simulink library "cm_custom"  (R2018b)
settings: Solver=VariableStepAuto  StartTime=0.0  StopTime=10.0  RelTol=1e-3
undefined symbols (not defined in the file or in its folder): DiscIntNeverNeededParam
libraries: simulink x19, raspberrypilib x4, $bdroot x2, speedgoatlib_fpga x2, androidcommunicationlib x1, embdlinuxlib x1, commutil2 x1
(part 1 of 2)
settings Model: Creator=carlosma  LastModifiedBy=Raymond
settings DebuggingCC: LibraryContextMissingDiagnostic=none
settings SFSimCC: SimUserLibraries=datatypes.h  SimUseLocalCustomCode=off
settings RTWCC: RTWUseLocalCustomCode=off  RTWUseSimCustomCode=on  CustomLibrary=datatypes.h  TargetLang=C++
settings GRTTargetCC: TargetLangStandard=C++03 (ISO)  MultiInstanceERTCode=on  CodeInterfacePackaging=C++ class

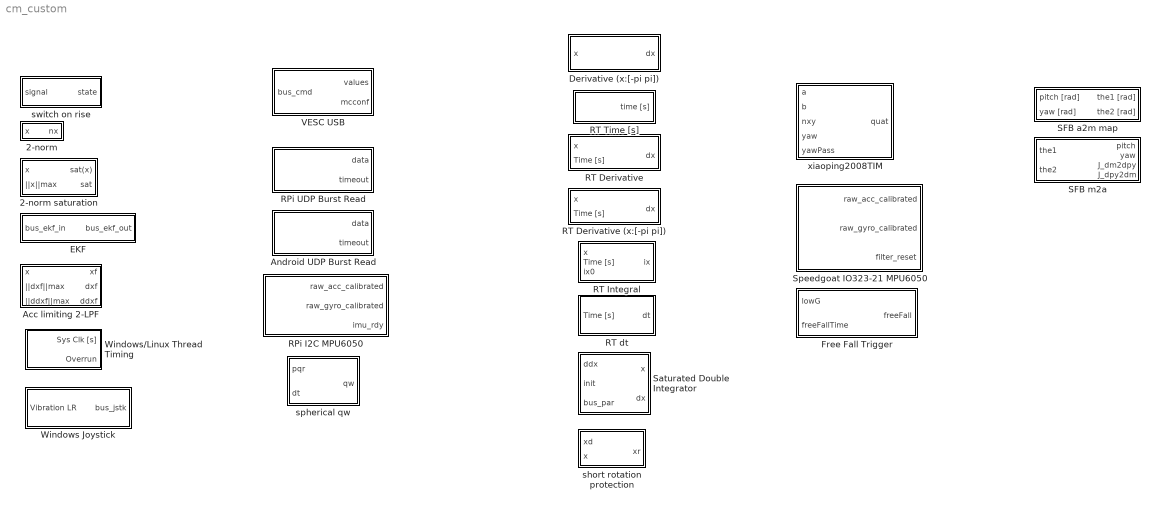
== system cm_custom ==
  2-norm : Subsystem  mask(Vector 2-norm){}
      mask help:
      | Computes vector 2-norm.
      |
      | ---
      | CMA 18DEC18
  2-norm saturation : Subsystem  mask(2-norm saturation){}
      mask help:
      | Saturates the input when its vector 2-norm reaches the defined limit.
      |
      | Maintains vector direction.
      |
      | ---
      | CMA 18DEC18
  Acc limiting 2-LPF : Subsystem  TreatAsAtomicUnit=on  SystemSampleTime=PAR_SMPLT  mask(Critically damped 2nd order LPF with acceleration and velocity limit){PAR_SMPLT=-1}
      mask prompts: PAR_SMPLT "Sampling Time [s]"
      mask help:
      | Limits are applied on the norms of the respective signals to retain signal directions.
      |
      | ddxf = -2*k*(xf - x) - k^2 * dxf;
      |
      | ||ddxf|| <= k^2 * ||xf - x|| + 2*k * ||dxf|| := ||ddxf||max
      | => k^2 * ||xf - x|| + k * 2 * ||dxf|| - ||ddxf||max = 0
      | => k = (-2*||dxf|| + sqrt(4*||dxf||^2 + 4 * ||xf - x|| * ||ddxf||max)) / (2 * ||xf - x|| + 1e-3); // norm division safe
      |
      | // satdxf not proven
  Android UDP Burst Read : Subsystem  TreatAsAtomicUnit=on  SystemSampleTime=PAR_SMPLT  mask(Android UDP Burst Read){PAR_LOCAL_IP_PORT=24001, PAR_BYTES_PER_PACKET=9, PAR_NBURST=100, PAR_TIMEOUT_TIME=1, PAR_SMPLT=0.1}
      mask prompts: PAR_LOCAL_IP_PORT "Local IP port"; PAR_BYTES_PER_PACKET "Expected nbytes per packet"; PAR_NBURST "Maximum burst read number"; PAR_TIMEOUT_TIME "Timeout after [s]"; PAR_SMPLT "Sampling Time [s]"
      mask help:
      | An extension to the official UDP read block.
      |
      | Supports burst reads and timeout detection.
      |
      | REQUIRES the official Simulink Android support package (2018b+).
      |
      | ---
      | Tested on a Samsung A9, Anrdroid 8.0.
      | Usable in External mode.
      | Embedded Coder safe.
      |
      | ---
      | CMA 8MAR2019
  Derivative (x:[-pi pi]) : Subsystem  TreatAsAtomicUnit=on  mask(RT Derivative (x:[-pi pi])){}
      mask help:
      | Computes the time derivative of the input using RT Time with x being an angular state between -pi and pi (matrix inputs are accepted).
      |
      | Requires one instance of the RT Time block.
      |
      | ---
      | Tested on Windows 10, Raspbian.
      | Usable in Simulation and External mode.
      | Embedded Coder safe.
      |
      | ---
      | CMA 14FEB19
  EKF : Subsystem  mask(EKF/LKF block){}
      mask help:
      | One step EKF computation for smooth nonlinear plants with continuous states.
      |
      | // Subscript 'o' means OLD
      | Smooth nonlinear plant with white process and measurement noises (wo, v)
      | x = f(xo, uo) + wo
      | y = g(x) + v
      |
      | bus_ekf_in signals
      | fuse // flag to activate or omit fusion
      | xh = f(xho, uo) // estimated mean
      | yh = g(xh) // estimated measurement
      | y // current measurement
      | A = df/dx | xo,uo // Jacobian A
      | B = df/du | xo,uo // Jacobian B
      | C = dg/dx | xh // Jacobian C
      | Qo = cov(wo) // process noise covariance
      | R = cov(v) // measurement noise covariance
      | Po = cov(xo-xho) // old mean covariance
      |
      | bus_ekf_out signals
      | x // filtered state mean
      | P // filtered state covariance
  Free Fall Trigger : Stateflow chart  TreatAsAtomicUnit=on
  RPi I2C MPU6050 : Stateflow chart  TreatAsAtomicUnit=on  SystemSampleTime=PAR_SMPLT  mask{PAR_SENS_ACC=([10.47 9.783 10.1] - [-9.234 -9.837 -9.396]) / 2 / 8192, PAR_SENS_GYRO=[1 1 1] * pi / 180 / 16.4, PAR_OFFSET_ACC=-[0.5758 -0.02694 0.673], PAR_OFFSET_GYRO=-[-0.133 -0.043 -0.023], PAR_SMPLT=0.001}
      mask prompts: PAR_SENS_ACC "Accelerometer sensitivities xyz [ms^-2/LSB]"; PAR_SENS_GYRO "Gyroscope sensitivities xyz [rad/LSB]"; PAR_OFFSET_ACC "Accelerometer offset xyz [ms^-2]"; PAR_OFFSET_GYRO "Gyroscope offset xyz [rad]"; PAR_SMPLT "Sampling Time [s]"
  RPi UDP Burst Read : Subsystem  TreatAsAtomicUnit=on  SystemSampleTime=PAR_SMPLT  mask(RPi UDP Burst Read){PAR_LOCAL_IP_PORT=24000, PAR_BYTES_PER_PACKET=13, PAR_NBURST=100, PAR_TIMEOUT_TIME=1, PAR_SMPLT=0.1}
      mask prompts: PAR_LOCAL_IP_PORT "Local IP port"; PAR_BYTES_PER_PACKET "Expected nbytes per packet"; PAR_NBURST "Maximum burst read number"; PAR_TIMEOUT_TIME "Timeout after [s]"; PAR_SMPLT "Sampling Time [s]"
      mask help:
      | An extension to the official UDP read block.
      |
      | Supports burst reads and timeout detection.
      |
      | REQUIRES the official Simulink Raspberry Pi support package (2018b+).
      |
      | ---
      | Tested on Raspbian.
      | Usable in External mode.
      | Embedded Coder safe.
      |
      | ---
      | CMA 8MAR2019
  RT Derivative : Subsystem  TreatAsAtomicUnit=on  mask(RT Derivative){}
      mask help:
      | Computes the time derivative of the input using RT Time.
      |
      | Requires one instance of the RT Time block.
      |
      | ---
      | Tested on Windows 10, Raspbian.
      | Usable in Simulation and External mode.
      | Embedded Coder safe.
      |
      | ---
      | CMA 14FEB19
  RT Derivative (x:[-pi pi]) : Subsystem  TreatAsAtomicUnit=on  mask(RT Derivative (x:[-pi pi])){}
      mask help:
      | Computes the time derivative of the input using RT Time with x being an angular state between -pi and pi (matrix inputs are accepted).
      |
      | Requires one instance of the RT Time block.
      |
      | ---
      | Tested on Windows 10, Raspbian.
      | Usable in Simulation and External mode.
      | Embedded Coder safe.
      |
      | ---
      | CMA 14FEB19
  RT Integral : Subsystem  TreatAsAtomicUnit=on  mask(RT Integral){PAR_SAT_UP=[inf], PAR_SAT_DOWN=[-inf]}
      mask prompts: PAR_SAT_UP "Upper integral saturation"; PAR_SAT_DOWN "Lower integral saturation"
      mask help:
      | Computes the time integral of the input using RT Time.
      |
      | Requires one instance of the RT Time block.
      |
      | ---
      | Tested on Windows 10, Raspbian.
      | Usable in Simulation and External mode.
      | Embedded Coder safe.
      |
      | ---
      | CMA 14FEB19
  RT Time [s] : Subsystem  mask(RT Time){}
      mask help:
      | Get RT time in seconds from <chrono>.
      |
      | ---
      | Tested on Windows 10, Raspbian.
      | Usable in Simulation.
      |
      | Link error on Windows external mode. - CMA 3APR19
      |
      | ---
      | CMA 3APR19
  RT dt : Subsystem  TreatAsAtomicUnit=on  mask(RT dt){}
      mask help:
      | Get last loop period using RT Time.
      |
      | Requires one instance of the RT Time block.
      |
      | ---
      | Tested on Windows 10, Raspbian.
      | Usable in Simulation and External mode.
      | Embedded Coder safe.
      |
      | ---
      | CMA 7MAR19
  SFB a2m map : Subsystem  mask(SFB M_a2m (YZX rotation)){par_r=0.05, par_w=0.05, par_yawMax=40*pi/180, par_pitchMax=90*pi/180}
      mask prompts: par_r "SFB bearing radius [m]"; par_w "SFB bearing width [m]"; par_yawMax "Maximum |yaw| [rad]"; par_pitchMax "Maximum |pitch| [rad]"
      mask help:
      | Maps yaw (psi) and pitch (the) angles of an SFB tail to the corresponding motor 1 and motor 2 angles.
      |
      | (Top view)
      |          T
      |          |
      |  M1   |    M2
      | (pitch up positive for both motors)
      |
      | thep = (the1 + the2) / 2;
      | thef = (the1 - the2) / 2;
      | the = thep;
      | tan(psi) = -2*r/w *sin(the_f);
      | |psi|_max = atan(2*r/w); // mechanical limit; will be used if superceded by the user limit
      |
      | ---
      | CMA 18DEC18
      mask init:
      | par_yawMax = min(par_yawMax, atan(2 * par_r / par_w));
  SFB m2a : MATLAB Function  TreatAsAtomicUnit=on
  Saturated Double Integrator : Subsystem  mask(Saturated Double Integrator){}
      mask help:
      | Second order integrator block with output and velocity saturations.
      |
      | ---
      | CMA 26MAR19
  Speedgoat IO323-21 MPU6050 : Stateflow chart  TreatAsAtomicUnit=on  SystemSampleTime=0.001  mask{PAR_SENS_ACC=[1 1 1] .* 9.80665 / 8192, PAR_SENS_GYRO=[1 1 1] * pi / 180 / 16.4, PAR_OFFSET_ACC=[-0.635 0.09 0.21], PAR_OFFSET_GYRO=[0.0462 0.0342 0.0261]}
      mask prompts: PAR_SENS_ACC "Accelerometer sensitivities xyz [ms^-2/LSB]"; PAR_SENS_GYRO "Gyroscope sensitivities xyz [rad/LSB]"; PAR_OFFSET_ACC "Accelerometer offset xyz [ms^-2]"; PAR_OFFSET_GYRO "Gyroscope offset xyz [rad]"
  VESC USB : Subsystem  InitFcn=load('vesc_usb_slx_buses.mat');  TreatAsAtomicUnit=on  SystemSampleTime=PAR_SMPLT  mask(VESC USB (Linux)){PAR_VESC_DEV='/dev/VESC_SFB_1', POS_KP=0.001, POS_KI=0, POS_KD=0.001, POS_KD_FIL=0.2, POS_DIV=1, CURR_MAX=20, CURR_MIN=-20, CURR_IN_MAX=20, CURR_IN_MIN=-20, CURR_ABS_MAX=20, PAR_SMPLT=0.05}
      mask prompts: PAR_VESC_DEV "VESC ID"; POS_KP "p_pid_kp"; POS_KI "p_pid_ki"; POS_KD "p_pid_kd"; POS_KD_FIL "p_pid_kd_filter"; POS_DIV "p_pid_ang_div"; CURR_MAX "l_current_max"; CURR_MIN "l_current_min"; CURR_IN_MAX "l_in_current_max"; CURR_IN_MIN "l_in_current_min"; CURR_ABS_MAX "l_abs_current_max"; PAR_SMPLT "Sampling Time [s]"
      mask help:
      | IO functions to and from a VESC via USB.
      | Drag and drop the same block for connecting to multiple VESC devices.
      |
      | --- SLX MASK
      | Allows the declaration of device name and R/W of some of the parameters of mcconfig.
      | ALWAYS READ mcconfig before WRITING.
      | Wrong mcconfig settings MAY DAMAGE your HW and brick your VESC.
      |
      | --- Compatible Firmware
      | 3.52, 3.53
      |
      | --- Compatible Hosts
      | Raspbian, Ubuntu 18.04.2 LTS.
      |
      | --- IO
      | bus_cmd: mode, pos_cmd, current_cmd
      | mode: [0 1 2 3 4] = [idle pos_PID read_mcconfig write_mcconfig current_ctrl]
      |
      | mc_values bus
      | mcconfig bus
      |
      | --- Fixing /DEV/ on Linux (assuming the device of interest is /dev/ttyUSB0)
      | CLI: udevadm info --name=/dev/ttyUSB0 --attribute-walk
      | mark down KERNEL and SUBSYSTEMS properties
      | e.g. KERNELS=="1-1.1.2", SUBSYSTEMS=="usb"
      | note that 1.1.2 in KERNELS means the second USB port
      | CLI: sudo nano /etc/udev/rules.d/99-USB_VESC.rules
      | add
      | KERNELS=="1-1.1.2", SUBSYSTEMS=="usb", SYMLINK+="VESC_SFB_1"
      | where "VESC_SFB_1" is the fixed desired USB device name.
      | Save, exit, reboot.
      | "VESC_SFB_1" is now fixed to USB port 2.
      |
      | ---
      | Usable in External mode.
      | Embedded Coder safe.
      |
      | ---
      | CMA 16MAY19
      mask init:
      | PAR_VESC_DEV = [PAR_VESC_DEV 0];
      mask DialogControl Control4 Prompt: mcconfig
      mask DialogControl Control2 Prompt: Fetch
      mask DialogControl Control2 Callback:
      | set_param(gcb+"/PAR_MASK_MODE", 'value', num2str(2));
      | 
      | rto = get_param(gcb+"/mcconfig_read_disp",'RuntimeObject');
      | while ~(rto.InputPort(1).Data(1))
      |     rto = get_param(gcb+"/mcconfig_read_disp",'RuntimeObject');
      |     pause(0.5);
      | end
      | 
      | rto = get_param(gcb+"/mcconfig_p_pid_disp",'RuntimeObject');
      | set_param(gcb, 'POS_KP', num2str(rto.InputPort(1).Data(1), 5));
      | set_param(gcb, 'POS_KI', num2str(rto.InputPort(1).Data(2), 5));
      | set_param(gcb, 'POS_KD', num2str(rto.InputPort(1).Data(3), 5));
      | set_param(gcb, 'POS_KD_FIL', num2str(rto.InputPort(1).Data(4), 5));
      | set_param(gcb, 'POS_DIV', num2str(rto.InputPort(1).Data(5), 5));
      | 
      | rto = get_param(gcb+"/mcconfig_current_lims_disp",'RuntimeObject');
      | set_param(gcb, 'CURR_MAX', num2str(rto.InputPort(1).Data(1), 5));
      | set_param(gcb, 'CURR_MIN', num2str(rto.InputPort(1).Data(2), 5));
      | set_param(gcb, 'CURR_IN_MAX', num2str(rto.InputPort(1).Data(3), 5));
      | set_param(gcb, 'CURR_IN_MIN', num2str(rto.InputPort(1).Data(4), 5));
      | set_param(gcb, 'CURR_ABS_MAX', num2str(rto.InputPort(1).Data(5), 5));
      | 
      | set_param(gcb+"/PAR_MASK_MODE", 'value', num2str(0));
      mask DialogControl Control3 Prompt: Write
      mask DialogControl Control3 Callback:
      | PID_PARAMS = [str2num(get_param(gcb, 'POS_KP')),...
      |               str2num(get_param(gcb, 'POS_KI')),...
      |               str2num(get_param(gcb, 'POS_KD')),...
      |               str2num(get_param(gcb, 'POS_KD_FIL')),...
      |               str2num(get_param(gcb, 'POS_DIV'))];
      | CURR_PARAMS = [str2num(get_param(gcb, 'CURR_MAX')),...
      |               str2num(get_param(gcb, 'CURR_MIN')),...
      |               str2num(get_param(gcb, 'CURR_IN_MAX')),...
      |               str2num(get_param(gcb, 'CURR_IN_MIN')),...
      |               str2num(get_param(gcb, 'CURR_ABS_MAX'))];
      | 
      | set_param(gcb+"/PAR_PID_GAINS", 'value', mat2str(PID_PARAMS));
      | set_param(gcb+"/PAR_CURR_LIMS", 'value', mat2str(CURR_PARAMS));
      | 
      | set_param(gcb+"/PAR_MASK_MODE", 'value', num2str(3)); % write mode
      | pause(0.5);
      | set_param(gcb+"/PAR_MASK_MODE", 'value', num2str(2)); % read mode
      | 
      | rto = get_param(gcb+"/mcconfig_read_disp",'RuntimeObject');
      | while ~(rto.InputPort(1).Data(1))
      |     rto = get_param(gcb+"/mcconfig_read_disp",'RuntimeObject');
      |     pause(0.5);
      | end
      | 
      | set_param(gcb+"/PAR_MASK_MODE", 'value', num2str(0));
  Windows Joystick : Subsystem  TreatAsAtomicUnit=on  SystemSampleTime=PAR_SMPLT  mask(Windows xinput joystick read){PAR_JSTKID=Joystick 1, PAR_SMPLT=0.05}
      mask prompts: PAR_JSTKID "Joystick ID"; PAR_SMPLT "Sampling Time [s]"
      mask help:
      | Tested on Windows 10 Enterprise Edition, x64, XBOX360 controller.
      | User can connect up to 4 controllers at the same time.
      |
      | This block can be used in both Normal and External modes.
      | Embedded Coder tolerant.
      |
      | Buttons [16]	[boolean]	[0 1]
      | LT RT 		[float] 		[-1 1]
      | LX LY RX RY	[float] 		[-1 1]
      | Connection 	[boolean]	[0 1]
      |
      | Vibration LR 	[float]		[0 1]
      |
      | ---
      | <windows.h>
      | <xinput.h>
      | #pragma comment(lib, "XInput.lib")
      |
      | ---
      | CMA 11DEC18
      mask init:
      | PAR_JSTKID = PAR_JSTKID - 1; % base zero
      mask TypeOptions PAR_JSTKID: Joystick 1 | Joystick 2 | Joystick 3 | Joystick 4
  Windows/Linux Thread Timing : Subsystem  TreatAsAtomicUnit=on  SystemSampleTime=PAR_SMPLT  mask(Thread Timing){PAR_SMPLT=1e-3}
      mask prompts: PAR_SMPLT "Thread base sampling time [s] (DO NOT USE -1)"
      mask help:
      | This block slows down the thread to close to real time.
      |
      | Tested on
      | - Windows 10 Enterprise Edition, x64,
      | - Ubuntu 18.04.2 LTS.
      |
      | This block can be used in both Normal and External Modes.
      |
      | Embedded Coder compatible.
      |
      | ---
      | #include<chrono>
      | #include<thread>
      |
      | ---
      | CMA 16MAY19
  short rotation protection : Subsystem  mask(Short Rotation Protection){PAR_MAX_XT=0.95*pi}
      mask prompts: PAR_MAX_XT "Maximum angular error (0,pi)"
      mask help:
      | This block ensures that the new commanded position will not cause an unwanted motor short rotation.
      |
      | The maximum angular error parameter X (<pi) ensures that the new reference angle would be at most X rad away from the current motor angle.
      |
      | e.g.
      | Without protection: if x = -150deg and xd = 150deg, a short short rotation of -60deg will occur downstream.
      | With protection: if x = -150deg and xd = 150deg, a proper rotation of +300deg will occur downstream.
      |
      | ---
      | CMA 26MAR19
  spherical qw : MATLAB Function  TreatAsAtomicUnit=on
  switch on rise : Subsystem  TreatAsAtomicUnit=on  mask(Switch on rise){}
      mask help: Toggles state (ON/OFF) on a rising edge of the input.
  xiaoping2008TIM : MATLAB Function  TreatAsAtomicUnit=on  SystemSampleTime=PAR_SMPLT  mask(Quaternion from accelerometer and magnetometer){PAR_SMPLT=-1}
      mask prompts: PAR_SMPLT "Sampling Time [s]"
      mask help: Quaternion from accelerometer and magnetometer

== system cm_custom/2-norm ==
  x : Inport
  Add : Sum  Inputs=+
  Sqrt : Sqrt  SaturateOnIntegerOverflow=on
  Square : Math  Operator=square  SaturateOnIntegerOverflow=on
  nx : Outport
  wires:
  Add/1 -> Sqrt/1
  Sqrt/1 -> nx/1
  Square/1 -> Add/1
  x/1 -> Square/1

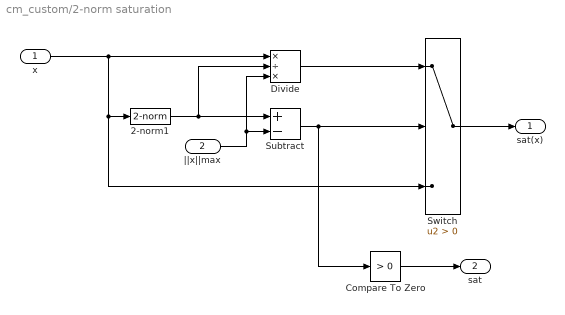
== system cm_custom/2-norm saturation ==
  x : Inport
  ||x||max : Inport  Port=2  PortDimensions=1
  2-norm1 : $bdroot/2-norm
  Compare To Zero : simulink/Logic and Bit Operations/Compare To Zero  relop=>  OutDataTypeStr=boolean
  Divide : Product  Inputs=*/*
  Subtract : Sum  Inputs=+-
  Switch : Switch  Criteria=u2 > Threshold
  sat(x) : Outport
  sat : Outport  Port=2
  wires:
  Compare To Zero/1 -> sat/1
  ||x||max/1 -> Divide/3, Subtract/2
  Subtract/1 -> Compare To Zero/1, Switch/2
  2-norm1/1 -> Divide/2, Subtract/1
  x/1 -> Switch/3, 2-norm1/1, Divide/1
  Switch/1 -> sat(x)/1
  Divide/1 -> Switch/1

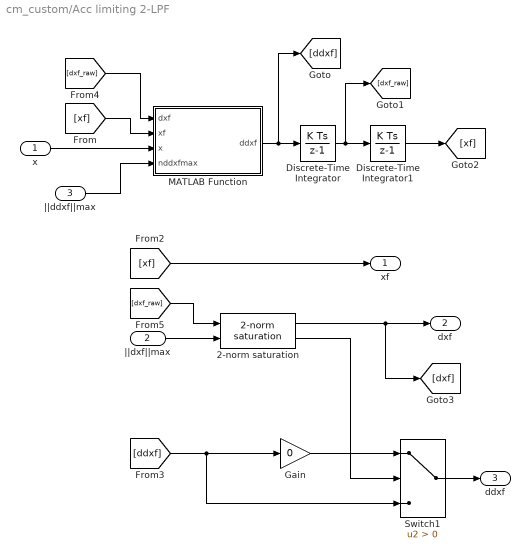
== system cm_custom/Acc limiting 2-LPF ==
  x : Inport
  ||dxf||max : Inport  Port=2
  ||ddxf||max : Inport  Port=3
  2-norm saturation : $bdroot/2-norm saturation
  Discrete-Time Integrator : DiscreteIntegrator  SampleTime=-1  ICPrevOutput=DiscIntNeverNeededParam  ICPrevScaledInput=DiscIntNeverNeededParam
  Discrete-Time Integrator1 : DiscreteIntegrator  SampleTime=-1  ICPrevOutput=DiscIntNeverNeededParam  ICPrevScaledInput=DiscIntNeverNeededParam
  Gain : Gain  Gain=0
  MATLAB Function : MATLAB Function
  Switch1 : Switch  Criteria=u2 > Threshold
  xf : Outport
  dxf : Outport  Port=2
  ddxf : Outport  Port=3
  wires:
  Discrete-Time Integrator/1 -> [dxf_raw], Discrete-Time Integrator1/1
  MATLAB Function/1(ddxf) -> Discrete-Time Integrator/1, [ddxf]
  x/1 -> MATLAB Function/3(x)
  ||ddxf||max/1 -> MATLAB Function/4(nddxfmax)
  Switch1/1 -> ddxf/1
  Gain/1 -> Switch1/1
  ||dxf||max/1 -> 2-norm saturation/2
  2-norm saturation/1 -> [dxf], dxf/1
  2-norm saturation/2 -> Switch1/2
  [xf] -> MATLAB Function/2(xf)
  [dxf_raw] -> MATLAB Function/1(dxf)
  Discrete-Time Integrator1/1 -> [xf]
  [xf] -> xf/1
  [ddxf] -> Switch1/3, Gain/1
  [dxf_raw] -> 2-norm saturation/1

== system cm_custom/Android UDP Burst Read ==
  Compare To Zero : simulink/Logic and Bit Operations/Compare To Zero  relop===  OutDataTypeStr=boolean
  Enabled Subsystem : Subsystem  TreatAsAtomicUnit=on
  Subsystem : Subsystem
  data : Outport
  timeout : Outport  Port=2
  wires:
  Enabled Subsystem/1(timeout) -> timeout/1  "timeout"
  Subsystem/2(nSuccessfulReads) -> Compare To Zero/1
  Compare To Zero/1 -> Enabled Subsystem/Enable
  Subsystem/1(data) -> data/1

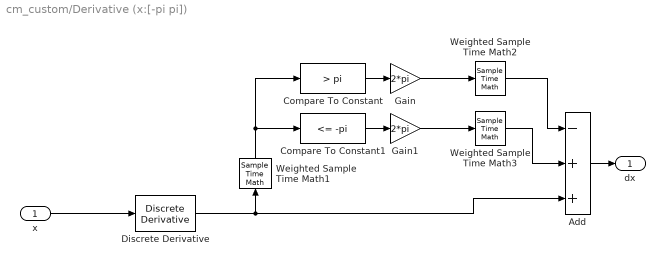
== system cm_custom/Derivative (x:[-pi pi]) ==
  x : Inport
  Add : Sum  Inputs=-++
  Compare To Constant : simulink/Logic and Bit Operations/Compare To Constant  relop=>  const=pi  OutDataTypeStr=boolean
  Compare To Constant1 : simulink/Logic and Bit Operations/Compare To Constant  relop=<=  const=-pi  OutDataTypeStr=boolean
  Discrete Derivative : simulink/Discrete/Discrete Derivative  gainval=1.0  ICPrevScaledInput=0.0  OutMin=[]  OutMax=[]  OutDataType=fixdt(1, 16)  OutScaling=2^-10  DoSatur=off
  Gain : Gain  Gain=2*pi  OutDataTypeStr=double
  Gain1 : Gain  Gain=2*pi  OutDataTypeStr=double
  Weighted Sample Time Math1 : SampleTimeMath  TsampMathOp=*
  Weighted Sample Time Math2 : SampleTimeMath  TsampMathOp=/
  Weighted Sample Time Math3 : SampleTimeMath  TsampMathOp=/
  dx : Outport
  wires:
  Discrete Derivative/1 -> Add/3, Weighted Sample Time Math1/1
  Compare To Constant/1 -> Gain/1
  Compare To Constant1/1 -> Gain1/1
  Gain/1 -> Weighted Sample Time Math2/1
  Gain1/1 -> Weighted Sample Time Math3/1
  x/1 -> Discrete Derivative/1
  Weighted Sample Time Math1/1 -> Compare To Constant/1, Compare To Constant1/1
  Weighted Sample Time Math2/1 -> Add/1
  Weighted Sample Time Math3/1 -> Add/2
  Add/1 -> dx/1

== system cm_custom/EKF ==
  bus_ekf_in : Inport
  Bus Creator1 : BusCreator  Inputs=2
  Bus Selector : BusSelector  OutputSignals=fuse,y,xh,yh,A,B,C,Qo,R,Po
  EKF : MATLAB Function  TreatAsAtomicUnit=on
  bus_ekf_out : Outport
  wires:
  Bus Selector/1 -> EKF/1(fuse)  "<fuse>"
  EKF/2(P) -> Bus Creator1/2  "P"
  Bus Selector/8 -> EKF/8(Qo)  "<Qo>"
  Bus Selector/6 -> EKF/6(B)  "<B>"
  Bus Creator1/1 -> bus_ekf_out/1  "bus_ekf_out"
  Bus Selector/5 -> EKF/5(A)  "<A>"
  Bus Selector/3 -> EKF/3(xh)  "<xh>"
  Bus Selector/4 -> EKF/4(yh)  "<yh>"
  Bus Selector/7 -> EKF/7(C)  "<C>"
  Bus Selector/9 -> EKF/9(R)  "<R>"
  EKF/1(x) -> Bus Creator1/1  "x"
  bus_ekf_in/1 -> Bus Selector/1  "bus_ekf_in"
  Bus Selector/2 -> EKF/2(y)  "<y>"
  Bus Selector/10 -> EKF/10(Po)  "<Po>"

== system cm_custom/RPi I2C MPU6050/initialization_sequence.reset.dev_reset ==
  f : TriggerPort  TriggerType=function-call  VariantControl=(inherit)
      settings: CopyFcn=Stateflow.SLINSF.SimulinkMan.removeBlockPreDeleteFcn  PreDeleteFcn=Stateflow.SLINSF.SimulinkMan.unsafePredeleteFcn
  Constant : Constant  Value=bin2dec('10000000')  OutDataTypeStr=uint8
  I2C Master Write : raspberrypilib/I2C Master Write  BoardProperty=Pi 3 Model B+  Mode=Master  SlaveAddress=hex2dec('68')  SlaveByteOrder=BigEndian  Direction=Transmitter  RegisterAddressMode=on  RegisterAddress=107  SlaveDataType=uint8  DataLength=1  NoAck=off  RepeatedStart=off  OutputStatus=on
      settings: SourceProductName=Simulink Support Package for Raspberry Pi Hardware  SourceProductBaseCode=RASPPI
  err : Outport
  wires:
  Constant/1 -> I2C Master Write/1
  I2C Master Write/1 -> err/1

== system cm_custom/RPi I2C MPU6050/initialization_sequence.settings.init_2 ==
  f : TriggerPort  TriggerType=function-call  VariantControl=(inherit)
      settings: CopyFcn=Stateflow.SLINSF.SimulinkMan.removeBlockPreDeleteFcn  PreDeleteFcn=Stateflow.SLINSF.SimulinkMan.unsafePredeleteFcn
  Constant : Constant  Value=0  OutDataTypeStr=uint8
  Constant1 : Constant  Value=0  OutDataTypeStr=uint8
  Constant2 : Constant  Value=bin2dec('00011000')  OutDataTypeStr=uint8
  Constant3 : Constant  Value=bin2dec('00001000')  OutDataTypeStr=uint8
  I2C Master Write : raspberrypilib/I2C Master Write  BoardProperty=Pi 3 Model B+  Mode=Master  SlaveAddress=hex2dec('68')  SlaveByteOrder=BigEndian  Direction=Transmitter  RegisterAddressMode=on  RegisterAddress=25  SlaveDataType=uint8  DataLength=1  NoAck=off  RepeatedStart=off  OutputStatus=on
      settings: SourceProductName=Simulink Support Package for Raspberry Pi Hardware  SourceProductBaseCode=RASPPI
  Mux : Mux
  err : Outport
  wires:
  Mux/1 -> I2C Master Write/1
  Constant3/1 -> Mux/4
  Constant/1 -> Mux/1
  Constant2/1 -> Mux/3
  Constant1/1 -> Mux/2
  I2C Master Write/1 -> err/1

== system cm_custom/RPi I2C MPU6050/initialization_sequence.wakeup.init_1 ==
  f : TriggerPort  TriggerType=function-call  VariantControl=(inherit)
      settings: CopyFcn=Stateflow.SLINSF.SimulinkMan.removeBlockPreDeleteFcn  PreDeleteFcn=Stateflow.SLINSF.SimulinkMan.unsafePredeleteFcn
  Constant : Constant  Value=bin2dec('00000001')  OutDataTypeStr=uint8
  I2C Master Write : raspberrypilib/I2C Master Write  BoardProperty=Pi 3 Model B+  Mode=Master  SlaveAddress=hex2dec('68')  SlaveByteOrder=BigEndian  Direction=Transmitter  RegisterAddressMode=on  RegisterAddress=107  SlaveDataType=uint8  DataLength=1  NoAck=off  RepeatedStart=off  OutputStatus=on
      settings: SourceProductName=Simulink Support Package for Raspberry Pi Hardware  SourceProductBaseCode=RASPPI
  err : Outport
  wires:
  Constant/1 -> I2C Master Write/1
  I2C Master Write/1 -> err/1

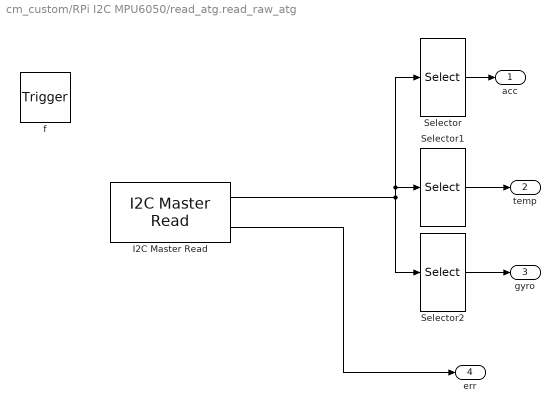
== system cm_custom/RPi I2C MPU6050/read_atg.read_raw_atg ==
  f : TriggerPort  TriggerType=function-call  VariantControl=(inherit)
      settings: CopyFcn=Stateflow.SLINSF.SimulinkMan.removeBlockPreDeleteFcn  PreDeleteFcn=Stateflow.SLINSF.SimulinkMan.unsafePredeleteFcn
  I2C Master Read : raspberrypilib/I2C Master Read  BoardProperty=Pi 3 Model B+  Mode=Master  SlaveAddress=hex2dec('68')  SlaveByteOrder=BigEndian  Direction=Receiver  RegisterAddressMode=on  RegisterAddress=59  SlaveDataType=int16  DataLength=7  NoAck=off  RepeatedStart=off  OutputStatus=on  SampleTime=-1
      settings: SourceProductName=Simulink Support Package for Raspberry Pi Hardware  SourceProductBaseCode=RASPPI
  Selector : Selector  InputPortWidth=7  IndexOptions=Index vector (dialog)  Indices=[1 2 3]  OutputSizes=1
  Selector1 : Selector  InputPortWidth=7  IndexOptions=Index vector (dialog)  Indices=4  OutputSizes=1
  Selector2 : Selector  InputPortWidth=7  IndexOptions=Index vector (dialog)  Indices=[5 6 7]  OutputSizes=1
  acc : Outport
  temp : Outport  Port=2
  gyro : Outport  Port=3
  err : Outport  Port=4  OutDataTypeStr=uint8
  wires:
  Selector2/1 -> gyro/1
  Selector1/1 -> temp/1
  Selector/1 -> acc/1
  I2C Master Read/2 -> err/1
  I2C Master Read/1 -> Selector2/1, Selector/1, Selector1/1

== system cm_custom/RPi UDP Burst Read ==
  Compare To Zero : simulink/Logic and Bit Operations/Compare To Zero  relop===  OutDataTypeStr=boolean
  Enabled Subsystem : Subsystem  TreatAsAtomicUnit=on
  Subsystem : Subsystem
  data : Outport
  timeout : Outport  Port=2
  wires:
  Enabled Subsystem/1(timeout) -> timeout/1  "timeout"
  Subsystem/2(nSuccessfulReads) -> Compare To Zero/1
  Compare To Zero/1 -> Enabled Subsystem/Enable
  Subsystem/1(data) -> data/1

== system cm_custom/RT Derivative ==
  x : Inport
  Time [s] : Inport  Port=2
  Delay : Delay  DelayLength=1
  Difference : simulink/Discrete/Difference  ICPrevInput=0.0  OutMin=[]  OutMax=[]  OutDataType=fixdt(1, 16)  OutScaling=2^-10  DoSatur=off
  Difference1 : simulink/Discrete/Difference  ICPrevInput=0.0  OutMin=[]  OutMax=[]  OutDataType=fixdt(1, 16)  OutScaling=2^-10  DoSatur=off
  Product : Product  Inputs=*/
  Switch : Switch  Criteria=u2 > Threshold
  dx : Outport
  wires:
  Difference/1 -> Product/1
  Difference1/1 -> Switch/2, Product/2
  Delay/1 -> Switch/3
  Switch/1 -> dx/1, Delay/1
  Product/1 -> Switch/1
  Time [s]/1 -> Difference1/1
  x/1 -> Difference/1

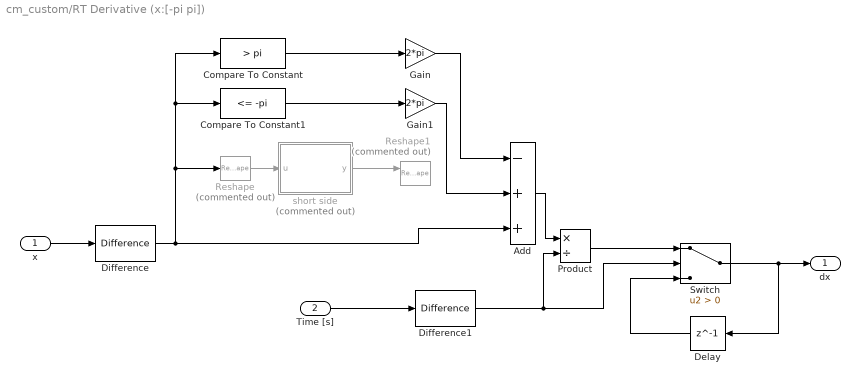
== system cm_custom/RT Derivative (x:[-pi pi]) ==
  x : Inport
  Time [s] : Inport  Port=2
  Add : Sum  Inputs=-++
  Compare To Constant : simulink/Logic and Bit Operations/Compare To Constant  relop=>  const=pi  OutDataTypeStr=boolean
  Compare To Constant1 : simulink/Logic and Bit Operations/Compare To Constant  relop=<=  const=-pi  OutDataTypeStr=boolean
  Delay : Delay  DelayLength=1
  Difference : simulink/Discrete/Difference  ICPrevInput=0.0  OutMin=[]  OutMax=[]  OutDataType=fixdt(1, 16)  OutScaling=2^-10  DoSatur=off
  Difference1 : simulink/Discrete/Difference  ICPrevInput=0.0  OutMin=[]  OutMax=[]  OutDataType=fixdt(1, 16)  OutScaling=2^-10  DoSatur=off
  Gain : Gain  Gain=2*pi  OutDataTypeStr=double
  Gain1 : Gain  Gain=2*pi  OutDataTypeStr=double
  Product : Product  Inputs=*/
  Reshape : Reshape  Commented=on
  Reshape1 : Reshape  Commented=on  OutputDimensionality=Derive from reference input port
  Switch : Switch  Criteria=u2 > Threshold
  short side : MATLAB Function  Commented=on  TreatAsAtomicUnit=on
  dx : Outport
  wires:
  short side/1(y) -> Reshape1/1
  Difference1/1 -> Switch/2, Product/2
  Reshape/1 -> short side/1(u)
  Difference/1 -> Add/3, Reshape/1, Compare To Constant1/1, Compare To Constant/1
  Delay/1 -> Switch/3
  Switch/1 -> dx/1, Delay/1
  Product/1 -> Switch/1
  Time [s]/1 -> Difference1/1
  x/1 -> Difference/1
  Compare To Constant/1 -> Gain/1
  Compare To Constant1/1 -> Gain1/1
  Add/1 -> Product/1
  Gain/1 -> Add/1
  Gain1/1 -> Add/2

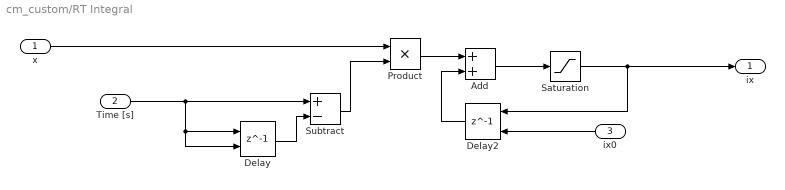
== system cm_custom/RT Integral ==
  x : Inport
  Time [s] : Inport  Port=2
  ix0 : Inport  Port=3
  Add : Sum
  Delay : Delay  DelayLength=1  InitialConditionSource=Input port
      settings: InputPortMap=u0,p4
  Delay2 : Delay  DelayLength=1  InitialConditionSource=Input port
      settings: InputPortMap=u0,p4
  Product : Product
  Saturation : Saturate  UpperLimit=PAR_SAT_UP  LowerLimit=PAR_SAT_DOWN
  Subtract : Sum  Inputs=+-
  ix : Outport
  wires:
  x/1 -> Product/1
  Delay2/1 -> Add/2
  Add/1 -> Saturation/1
  Subtract/1 -> Product/2
  Time [s]/1 -> Delay/1, Delay/2, Subtract/1
  Delay/1 -> Subtract/2
  Product/1 -> Add/1
  Saturation/1 -> ix/1, Delay2/1
  ix0/1 -> Delay2/2

== system cm_custom/RT Time [s] ==
  S-Function Builder : S-Function  InitFcn=try, set_param(gcb,'FunctionName','sf_chrono_getCpuTime_secs'), end  FunctionName=sf_chrono_getCpuTime_secs  SFunctionModules=sf_chrono_getCpuTime_secs_wrapper  SFunctionDeploymentMode=off  EnableBusSupport=off  mask(S-Function Builder){}
      mask help: Simulink:masks:SFunctionBuilder_MD
      mask init:
      | val = [[.9  0.75 0.75 1 1 .9 .9 1]',[1 1 0.75 0.75 .9 .9 1 .9]'];try , sys = get_param(gcb,'SfunBuilderFcnName');if isempty(sys), sys = get_param(gcb,'FunctionName'); end,catch, sys = get_param(gcb,'FunctionName'); end
      settings: CopyFcn=set_param(gcbh,'LinkStatus','none')  PreSaveFcn=try, set_param(gcb,'FunctionName','sf_chrono_getCpuTime_secs'), end  OpenFcn=sfunctionwizard(gcbh)
      mask Display: plot(val(:,1),val(:,2)),disp(sys), port_label('output',1,'slx_secs')
  time [s] : Outport
  wires:
  S-Function Builder/1 -> time [s]/1

== system cm_custom/RT dt ==
  Time [s] : Inport
  Difference : simulink/Discrete/Difference  ICPrevInput=0.0  OutMin=[]  OutMax=[]  OutDataType=fixdt(1, 16)  OutScaling=2^-10  DoSatur=off
  dt : Outport
  wires:
  Time [s]/1 -> Difference/1
  Difference/1 -> dt/1

== system cm_custom/SFB a2m map ==
  pitch [rad] : Inport
  yaw [rad] : Inport  Port=2
  M_a2m : MATLAB Function  TreatAsAtomicUnit=on
  the1 [rad] : Outport
  the2 [rad] : Outport  Port=2
  wires:
  M_a2m/2(the2) -> the2 [rad]/1
  M_a2m/1(the1) -> the1 [rad]/1
  pitch [rad]/1 -> M_a2m/2(the)
  yaw [rad]/1 -> M_a2m/1(psi)

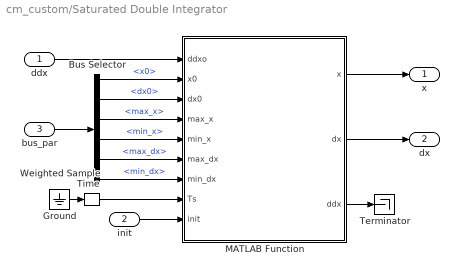
== system cm_custom/Saturated Double Integrator ==
  ddx : Inport
  init : Inport  Port=2
  bus_par : Inport  Port=3
  Bus Selector : BusSelector  OutputSignals=x0,dx0,max_x,min_x,max_dx,min_dx
  Ground : Ground
  MATLAB Function : MATLAB Function  TreatAsAtomicUnit=on
  Terminator : Terminator
  Weighted Sample Time : SampleTimeMath  TsampMathOp=Ts Only
  x : Outport
  dx : Outport  Port=2
  wires:
  MATLAB Function/1(x) -> x/1
  ddx/1 -> MATLAB Function/1(ddxo)
  bus_par/1 -> Bus Selector/1
  init/1 -> MATLAB Function/9(init)
  MATLAB Function/3(ddx) -> Terminator/1
  MATLAB Function/2(dx) -> dx/1
  Weighted Sample Time/1 -> MATLAB Function/8(Ts)
  Ground/1 -> Weighted Sample Time/1
  Bus Selector/3 -> MATLAB Function/4(max_x)  "<max_x>"
  Bus Selector/2 -> MATLAB Function/3(dx0)  "<dx0>"
  Bus Selector/4 -> MATLAB Function/5(min_x)  "<min_x>"
  Bus Selector/1 -> MATLAB Function/2(x0)  "<x0>"
  Bus Selector/5 -> MATLAB Function/6(max_dx)  "<max_dx>"
  Bus Selector/6 -> MATLAB Function/7(min_dx)  "<min_dx>"

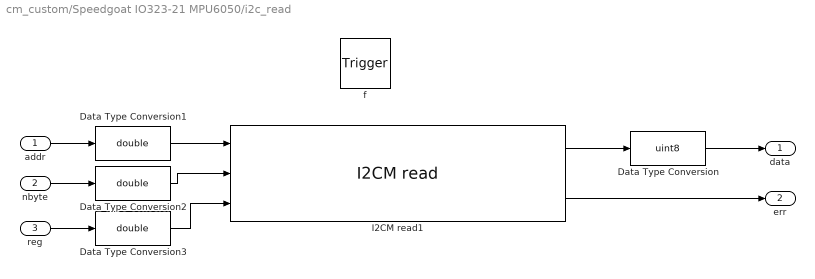
== system cm_custom/Speedgoat IO323-21 MPU6050/i2c_read ==
  addr : Inport  OutDataTypeStr=uint8  PortDimensions=1
  nbyte : Inport  Port=2  OutDataTypeStr=uint8  PortDimensions=1
  reg : Inport  Port=3  OutDataTypeStr=uint8  PortDimensions=1
  f : TriggerPort  TriggerType=function-call  VariantControl=(inherit)
      settings: CopyFcn=Stateflow.SLINSF.SimulinkMan.removeBlockPreDeleteFcn  PreDeleteFcn=Stateflow.SLINSF.SimulinkMan.unsafePredeleteFcn
  Data Type Conversion : DataTypeConversion  OutDataTypeStr=uint8
  Data Type Conversion1 : DataTypeConversion  OutDataTypeStr=double
  Data Type Conversion2 : DataTypeConversion  OutDataTypeStr=double
  Data Type Conversion3 : DataTypeConversion  OutDataTypeStr=double
  I2CM read1 : speedgoatlib_fpga/I2C/I2CM read  id=1  chan=1  ts=-1  pciSlot=-1  board=Please select...  clockDivider=375/4  subIndexConfiguration=on  showAckErrorPort=on
      settings: SourceProductName=Simulink Real-Time: Speedgoat I/O Driver Library
  data : Outport
  err : Outport  Port=2  OutDataTypeStr=boolean
  wires:
  addr/1 -> Data Type Conversion1/1
  nbyte/1 -> Data Type Conversion2/1
  I2CM read1/2 -> err/1
  I2CM read1/1 -> Data Type Conversion/1
  Data Type Conversion1/1 -> I2CM read1/1
  Data Type Conversion2/1 -> I2CM read1/2
  reg/1 -> Data Type Conversion3/1
  Data Type Conversion3/1 -> I2CM read1/3
  Data Type Conversion/1 -> data/1

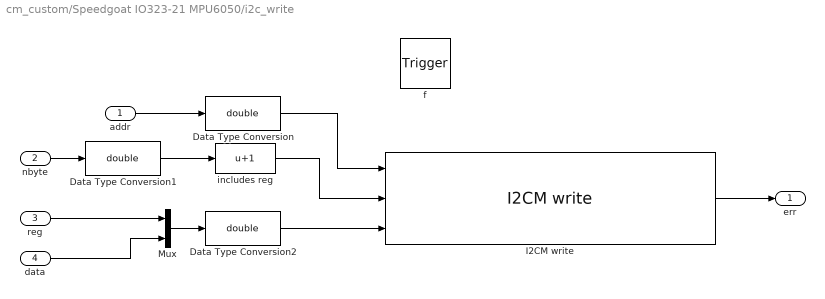
== system cm_custom/Speedgoat IO323-21 MPU6050/i2c_write ==
  addr : Inport  OutDataTypeStr=uint8  PortDimensions=1
  nbyte : Inport  Port=2  OutDataTypeStr=uint8  PortDimensions=1
  reg : Inport  Port=3  OutDataTypeStr=uint8  PortDimensions=1
  data : Inport  Port=4  OutDataTypeStr=uint8  PortDimensions=63
  f : TriggerPort  TriggerType=function-call  VariantControl=(inherit)
      settings: CopyFcn=Stateflow.SLINSF.SimulinkMan.removeBlockPreDeleteFcn  PreDeleteFcn=Stateflow.SLINSF.SimulinkMan.unsafePredeleteFcn
  Data Type Conversion : DataTypeConversion  OutDataTypeStr=double
  Data Type Conversion1 : DataTypeConversion  OutDataTypeStr=double
  Data Type Conversion2 : DataTypeConversion  OutDataTypeStr=double
  I2CM write : speedgoatlib_fpga/I2C/I2CM write  id=1  chan=1  ts=-1  pciSlot=-1  board=Please select...  clockDivider=375/4  showAckErrorPort=on
      settings: SourceProductName=Simulink Real-Time: Speedgoat I/O Driver Library
  Mux : Mux  Inputs=2
  includes reg : Fcn  Expr=u+1
  err : Outport
  wires:
  addr/1 -> Data Type Conversion/1
  nbyte/1 -> Data Type Conversion1/1
  data/1 -> Mux/2
  reg/1 -> Mux/1
  Mux/1 -> Data Type Conversion2/1
  I2CM write/1 -> err/1
  Data Type Conversion/1 -> I2CM write/1
  Data Type Conversion1/1 -> includes reg/1
  Data Type Conversion2/1 -> I2CM write/3
  includes reg/1 -> I2CM write/2

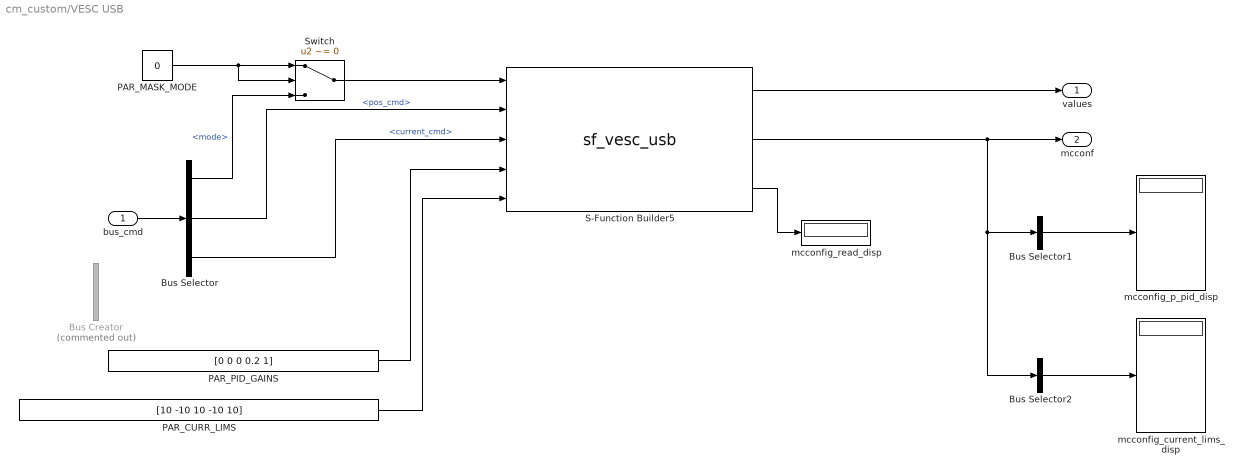
== system cm_custom/VESC USB ==
  bus_cmd : Inport
  Bus Creator : BusCreator  Commented=on  Inputs=3
  Bus Selector : BusSelector  OutputSignals=mode,pos_cmd,current_cmd
  Bus Selector1 : BusSelector  OutputSignals=p_pid_kp,p_pid_ki,p_pid_kd,p_pid_kd_filter,p_pid_ang_div  OutputAsBus=on
  Bus Selector2 : BusSelector  OutputSignals=l_current_max,l_current_min,l_in_current_max,l_in_current_min,l_abs_current_max  OutputAsBus=on
  PAR_CURR_LIMS : Constant  Value=[10 -10 10 -10 10]
  PAR_MASK_MODE : Constant  Value=0  OutDataTypeStr=uint32
  PAR_PID_GAINS : Constant  Value=[0 0 0 0.2 1]
  S-Function Builder5 : S-Function  InitFcn=try, set_param(gcb,'FunctionName','sf_vesc_usb'), end  FunctionName=sf_vesc_usb  Parameters=uint8(PAR_VESC_DEV)  SFunctionModules=sf_vesc_usb_wrapper  SFunctionDeploymentMode=off  EnableBusSupport=off  mask(S-Function Builder){}
      mask help: Simulink:masks:SFunctionBuilder_MD
      mask init: same as cm_custom/RT Time [s]/S-Function Builder
      settings: CopyFcn=set_param(gcbh,'LinkStatus','none')  PreSaveFcn=try, set_param(gcb,'FunctionName','sf_vesc_usb'), end  OpenFcn=sfunctionwizard(gcbh)
      mask Display: plot(val(:,1),val(:,2)),disp(sys), port_label('input',1,'slx_mode'), port_label('input',2,'slx_pos_cmd'), port_label('input',3,'slx_current_cmd'), port_label('input',4,'slx_pos_pid_gains'), port_label('input',5,'slx_curr_lims'), port_label('output',1,'slx_values'), port_label('output',2,'slx_mcconf'), port_label('output',3,'slx_mcconf_read')
  Switch : Switch  Criteria=u2 ~= 0
  mcconfig_current_lims_disp : Display
  mcconfig_p_pid_disp : Display
  mcconfig_read_disp : Display
  values : Outport  OutDataTypeStr=Bus: mc_values
  mcconf : Outport  Port=2  OutDataTypeStr=Bus: mc_configuration
  wires:
  S-Function Builder5/2 -> Bus Selector2/1, Bus Selector1/1, mcconf/1
  S-Function Builder5/1 -> values/1
  PAR_PID_GAINS/1 -> S-Function Builder5/4
  Bus Selector1/1 -> mcconfig_p_pid_disp/1
  Bus Selector2/1 -> mcconfig_current_lims_disp/1
  PAR_CURR_LIMS/1 -> S-Function Builder5/5
  PAR_MASK_MODE/1 -> Switch/2, Switch/1
  Switch/1 -> S-Function Builder5/1
  S-Function Builder5/3 -> mcconfig_read_disp/1
  bus_cmd/1 -> Bus Selector/1
  Bus Selector/1 -> Switch/3  "<mode>"
  Bus Selector/2 -> S-Function Builder5/2  "<pos_cmd>"
  Bus Selector/3 -> S-Function Builder5/3  "<current_cmd>"
  ? -> Bus Creator/2  "pos_cmd"
  ? -> Bus Creator/1  "mode"
  ? -> Bus Creator/3  "current_cmd"

== system cm_custom/Windows Joystick ==
  Vibration LR : Inport
  Bus Creator : BusCreator  Inputs=8
  Demux : Demux  Outputs=2
  Integer to Bit Converter : commutil2/Integer to Bit Converter  nbits=16  signedInputValues=Unsigned  bitOrder=MSB first  outDtype=boolean
      settings: SourceProductName=Communications Toolbox
  S-Function Builder : S-Function  InitFcn=try, set_param(gcb,'FunctionName','sf_windows_xinput_jstk'), end  FunctionName=sf_windows_xinput_jstk  Parameters=uint8(PAR_JSTKID)  SFunctionModules=sf_windows_xinput_jstk_wrapper  SFunctionDeploymentMode=off  EnableBusSupport=off  mask(S-Function Builder){}
      mask help: Simulink:masks:SFunctionBuilder_MD
      mask init: same as cm_custom/RT Time [s]/S-Function Builder
      settings: CopyFcn=set_param(gcbh,'LinkStatus','none')  PreSaveFcn=try, set_param(gcb,'FunctionName','sf_windows_xinput_jstk'), end  OpenFcn=sfunctionwizard(gcbh)
      mask Display: plot(val(:,1),val(:,2)),disp(sys), port_label('input',1,'wLeftMotorSpeed'), port_label('input',2,'wRightMotorSpeed'), port_label('output',1,'wButtons'), port_label('output',2,'bLeftTrigger'), port_label('output',3,'bRightTrigger'), port_label('output',4,'sThumbLX'), port_label('output',5,'sThumbLY'), port_label('output',6,'sThumbRX'), port_label('output',7,'sThumbRY'), port_label('output',8,'jstkConnected')
  Saturation : Saturate  UpperLimit=1  LowerLimit=0
  bus_jstk : Outport
  wires:
  S-Function Builder/1 -> Integer to Bit Converter/1
  Integer to Bit Converter/1 -> Bus Creator/1  "buttons"
  S-Function Builder/2 -> Bus Creator/2  "LT"
  S-Function Builder/3 -> Bus Creator/3  "RT"
  S-Function Builder/4 -> Bus Creator/4  "LX"
  S-Function Builder/5 -> Bus Creator/5  "LY"
  S-Function Builder/6 -> Bus Creator/6  "RX"
  S-Function Builder/7 -> Bus Creator/7  "RY"
  S-Function Builder/8 -> Bus Creator/8  "Connection"
  Bus Creator/1 -> bus_jstk/1
  Vibration LR/1 -> Saturation/1
  Demux/1 -> S-Function Builder/1
  Demux/2 -> S-Function Builder/2
  Saturation/1 -> Demux/1

== system cm_custom/Windows//Linux Thread Timing ==
  Compare To Zero : simulink/Logic and Bit Operations/Compare To Zero  relop=<  OutDataTypeStr=boolean
  S-Function Builder : S-Function  InitFcn=try, set_param(gcb,'FunctionName','sf_chrono_thread'), end  FunctionName=sf_chrono_thread  Parameters=PAR_SMPLT  SFunctionModules=sf_chrono_thread_wrapper  SFunctionDeploymentMode=off  EnableBusSupport=off  mask(S-Function Builder){}
      mask help: Simulink:masks:SFunctionBuilder_MD
      mask init: same as cm_custom/RT Time [s]/S-Function Builder
      settings: CopyFcn=set_param(gcbh,'LinkStatus','none')  PreSaveFcn=try, set_param(gcb,'FunctionName','sf_chrono_thread'), end  OpenFcn=sfunctionwizard(gcbh)
      mask Display: plot(val(:,1),val(:,2)),disp(sys), port_label('output',1,'sys_clock_s'), port_label('output',2,'loop_time_left_s')
  Sys Clk [s] : Outport
  Overrun : Outport  Port=2
  wires:
  S-Function Builder/2 -> Compare To Zero/1
  S-Function Builder/1 -> Sys Clk [s]/1
  Compare To Zero/1 -> Overrun/1

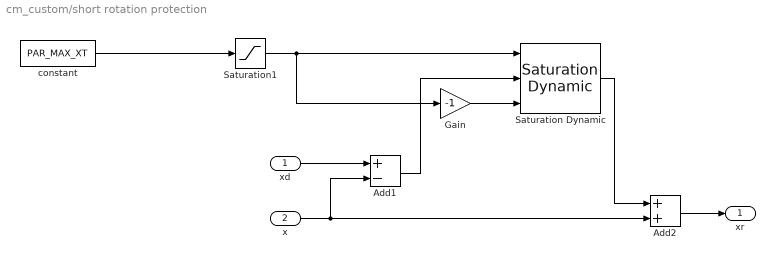
== system cm_custom/short rotation protection ==
  xd : Inport
  x : Inport  Port=2
  Add1 : Sum  Inputs=+-
  Add2 : Sum
  Gain : Gain  Gain=-1
  Saturation Dynamic : simulink/Discontinuities/Saturation Dynamic  OutMin=[]  OutMax=[]  OutDataTypeStr=Inherit: Same as second input  OutDataType=fixdt(1, 16)  OutScaling=2^-10  DoSatur=off
  Saturation1 : Saturate  UpperLimit=pi  LowerLimit=0
  "constant " : Constant  Value=PAR_MAX_XT
  xr : Outport
  wires:
  "constant "/1 -> Saturation1/1
  Add1/1 -> Saturation Dynamic/2
  Gain/1 -> Saturation Dynamic/3
  Saturation1/1 -> Saturation Dynamic/1, Gain/1
  Saturation Dynamic/1 -> Add2/1
  Add2/1 -> xr/1
  x/1 -> Add2/2, Add1/2
  xd/1 -> Add1/1

== system cm_custom/switch on rise ==
  signal : Inport
  Subsystem : Subsystem
  state : Outport
  wires:
  Subsystem/1(state) -> state/1
  signal/1 -> Subsystem/Trigger

== system cm_custom/Android UDP Burst Read/Enabled Subsystem ==
  Enable : EnablePort  StatesWhenEnabling=reset
  Compare To Constant : simulink/Logic and Bit Operations/Compare To Constant  relop=>=  const=PAR_TIMEOUT_TIME  OutDataTypeStr=boolean
  Constant : Constant
  Discrete-Time Integrator : DiscreteIntegrator  SampleTime=-1  ICPrevOutput=DiscIntNeverNeededParam  ICPrevScaledInput=DiscIntNeverNeededParam
  timeout : Outport  OutputWhenDisabled=reset  InitialOutput=0
  wires:
  Compare To Constant/1 -> timeout/1
  Constant/1 -> Discrete-Time Integrator/1
  Discrete-Time Integrator/1 -> Compare To Constant/1

== system cm_custom/Android UDP Burst Read/Subsystem ==
  Compare To Constant : simulink/Logic and Bit Operations/Compare To Constant  relop===  const=PAR_BYTES_PER_PACKET  OutDataTypeStr=boolean
  Constant : Constant
  Subtract : Sum  Inputs=+-
  UDP Receive1 : androidcommunicationlib/UDP Receive  localURL='0.0.0.0'  localPort=PAR_LOCAL_IP_PORT  remoteURL='0.0.0.0'  remotePort=-1  recvBufferSize=8192  signalDatatype=uint8  dims=PAR_BYTES_PER_PACKET  isVarSize=off  showBlockingTime=off  blockingTime=0  sampletime=-1  blockPlatform=Android
      settings: SourceProductName=Simulink Support Package for Android Devices  SourceProductBaseCode=ANDROID
  While Iterator : WhileIterator  MaxIters=PAR_NBURST  WhileBlockType=do-while  ShowIterationPort=on  OutputDataType=double
  data : Outport
  nSuccessfulReads : Outport  Port=2
  wires:
  Subtract/1 -> nSuccessfulReads/1
  Constant/1 -> Subtract/2
  While Iterator/1 -> Subtract/1
  Compare To Constant/1 -> While Iterator/1
  UDP Receive1/1 -> data/1
  UDP Receive1/2 -> Compare To Constant/1

== system cm_custom/RPi UDP Burst Read/Enabled Subsystem ==
  Enable : EnablePort  StatesWhenEnabling=reset
  Compare To Constant : simulink/Logic and Bit Operations/Compare To Constant  relop=>=  const=PAR_TIMEOUT_TIME  OutDataTypeStr=boolean
  Constant : Constant
  Discrete-Time Integrator : DiscreteIntegrator  SampleTime=-1  ICPrevOutput=DiscIntNeverNeededParam  ICPrevScaledInput=DiscIntNeverNeededParam
  timeout : Outport  OutputWhenDisabled=reset  InitialOutput=0
  wires:
  Compare To Constant/1 -> timeout/1
  Constant/1 -> Discrete-Time Integrator/1
  Discrete-Time Integrator/1 -> Compare To Constant/1

== system cm_custom/RPi UDP Burst Read/Subsystem ==
  Compare To Constant : simulink/Logic and Bit Operations/Compare To Constant  relop===  const=PAR_BYTES_PER_PACKET  OutDataTypeStr=boolean
  Constant : Constant
  Subtract : Sum  Inputs=+-
  UDP Receive : embdlinuxlib/UDP Receive  localURL='0.0.0.0'  localPort=PAR_LOCAL_IP_PORT  remoteURL='0.0.0.0'  remotePort=-1  recvBufferSize=8192  signalDatatype=uint8  dims=PAR_BYTES_PER_PACKET  isVarSize=off  showBlockingTime=off  blockingTime=0  sampletime=-1  blockPlatform=Raspberry Pi
      settings: SourceProductName=Simulink Support Package for Raspberry Pi Hardware  SourceProductBaseCode=RASPPI
  While Iterator : WhileIterator  MaxIters=PAR_NBURST  WhileBlockType=do-while  ShowIterationPort=on  OutputDataType=double
  data : Outport
  nSuccessfulReads : Outport  Port=2
  wires:
  Subtract/1 -> nSuccessfulReads/1
  Constant/1 -> Subtract/2
  While Iterator/1 -> Subtract/1
  Compare To Constant/1 -> While Iterator/1
  UDP Receive/1 -> data/1
  UDP Receive/2 -> Compare To Constant/1

== system cm_custom/switch on rise/Subsystem ==
  Trigger : TriggerPort  VariantControl=Variant  PortDimensions=1
  Delay : Delay  DelayLength=1  InitialCondition=boolean(1)
  NOT : Logic  Operator=NOT  AllPortsSameDT=off  OutDataTypeStr=boolean
  state : Outport
  wires:
  NOT/1 -> state/1, Delay/1
  Delay/1 -> NOT/1

== matlab function cm_custom/xiaoping2008TIM ==
  data: a input; quat output; b input; nxy input; yaw input; yawPass input
function quat = accMag2Quat(a, b, nxy, yaw, yawPass)
%#codegen
%% init
quat = [1 0 0 0]';
qp = [1 0 0 0];
qr = [1 0 0 0];
qy = [1 0 0 0];

aNorm = (a(1)^2 + a(2)^2 + a(3)^2) ^ 0.5;

if aNorm > 1e-3 
    a = a ./ aNorm;
    
    %% pitch
    sp = a(1);
    cp = (1 - sp ^ 2) ^ 0.5;
    spb2 = sign(sp) * ((1 - cp) / 2) ^ 0.5;
    cpb2 = ((1 + cp) / 2) ^ 0.5;
    qp = [cpb2 0 spb2 0]; 
    
    %% roll
    if (cp < 1e-3)
        qr = [1 0 0 0];
    else
        sr = -a(2) / cp;
        cr = -a(3) / cp;
        if (cr == -1 && sr == 0)
            qr = [0 ((1 - cr) / 2) ^ 0.5 0 0];
        else
            srb2 = sign(sr) * ((1 - cr) / 2) ^ 0.5;
            crb2 = ((1 + cr) / 2) ^ 0.5;
            qr = [crb2 srb2 0 0];
        end
    end
    
    %% yaw
    
    if ~yawPass
        b = b ./ (b(1) ^ 2 + b(2) ^ 2 + b(3) ^ 2) ^ 0.5;
        qb = [0 0 0 0];
        qb = [0 b'];
        qb = quatmultiply(qr, quatmultiply(qb, quatconj(qr)));
        qb = quatmultiply(qp, quatmultiply(qb, quatconj(qp)));
        
        cb = qb(2:4);
        ncb = (cb(1) ^ 2 + cb(2) ^ 2) ^ 0.5;
        mxy = [0 0];
        if ncb > 0
            mxy = cb(1:2) ./ ncb;
        end
        
        csy = [mxy(1) mxy(2); -mxy(2) mxy(1)] * nxy;
        
        
        syb2 = sign(csy(2)) * ((1 - csy(1)) / 2) ^ 0.5;
        cyb2 = ((1 + csy(1)) / 2) ^ 0.5;
        if syb2 ~= 0 && cyb2 ~= 0
            qy = [cyb2 0 0 syb2];
        end
    else
        qy = [cos(yaw/2) 0 0 sin(yaw/2)];
    end
    
    quat = quatmultiply(qy, quatmultiply(qp, qr))';
    
end

== matlab function cm_custom/Acc limiting 2-LPF/MATLAB Function ==
  data: dxf input; ddxf output; xf input; x input; nddxfmax input size=1
function ddxf = acclim_2lpf(dxf, xf, x, nddxfmax)

xft = xf - x;
nxft = (sum(xft.^2))^0.5;
ndxf = (sum(dxf.^2))^0.5;

k = (-2*ndxf + sqrt(4*ndxf^2 + 4*nxft*nddxfmax)) / (2*nxft + 1e-3);

ddxf = -k^2 * xft - 2*k*dxf;

== stateflow chart cm_custom/Speedgoat IO323-21 MPU6050 ==
  state initialization_sequence
    state settings
      entry:
      // SMPRT_DIV, CONFIG, GYRO_CONFIG, ACCEL_CONFIG
      write_buffer[0] = 0; // full hardware sampling rate
      write_buffer[1] = 0; // no sync, no LP
      write_buffer[2] = 3 << 3; // +- 2000dps
      write_buffer[3] = 1 << 3; // +- 4g
      i2c_write(0x68, 4, 25, write_buffer);
    state wakeup
      entry:
      filter_reset = false;
      // PWR_MGMT_1
      //write_buffer[0] = 1 << 7; // reset
      //i2c_write(0x68, 1, 107, write_buffer);
      // PWR_MGMT_1
      write_buffer[0] = (0 << 6) | (1 << 0); // wake up, gyro clock
      i2c_write(0x68, 1, 107, write_buffer);
    (default) -> wakeup
    wakeup -> settings : after(0.2, sec)
  state err = i2c_write(addr,nbyte,reg,data) [function]
  state [data,err] = i2c_read(addr,nbyte,reg) [function]
  state read_atg
    entry:
    filter_reset = true;
    during:
    // WHO AM I
    //[read_buffer, read_err] = i2c_read(0x68, 1, 117);
    //who_am_i = read_buffer[0];
    // ACCEL, TEMP, GYRO OUT
    [read_buffer, read_err] = i2c_read(0x68, 14, 59);
    raw_acc[0] = int16(read_buffer[0] << 8 | read_buffer[1]);
    raw_acc[1] = int16(read_buffer[2] << 8 | read_buffer[3]);
    raw_acc[2] = int16(read_buffer[4] << 8 | read_buffer[5]);
    raw_temp = int16(read_buffer[6] << 8 | read_buffer[7]);
    raw_gyro[0] = int16(read_buffer[8] << 8 | read_buffer[9]);
    raw_gyro[1] = int16(read_buffer[10] << 8 | read_buffer[11]);
    raw_gyro[2] = int16(read_buffer[12] << 8 | read_buffer[13]);
    // offset sensitivities
    raw_acc_calibrated[0] = (double(raw_acc[0]) * PAR_SENS_ACC[0]) + PAR_OFFSET_ACC[0];
    raw_acc_calibrated[1] = (double(raw_acc[1]) * PAR_SENS_ACC[1]) + PAR_OFFSET_ACC[1];
    raw_acc_calibrated[2] = (double(raw_acc[2]) * PAR_SENS_ACC[2]) + PAR_OFFSET_ACC[2];
    raw_gyro_calibrated[0] = (double(raw_gyro[0]) * PAR_SENS_GYRO[0]) + PAR_OFFSET_GYRO[0];
    raw_gyro_calibrated[1] = (double(raw_gyro[1]) * PAR_SENS_GYRO[1]) + PAR_OFFSET_GYRO[1];
    raw_gyro_calibrated[2] = (double(raw_gyro[2]) * PAR_SENS_GYRO[2]) + PAR_OFFSET_GYRO[2];
  (default) -> initialization_sequence
  initialization_sequence -> read_atg : after(1, sec)
  data: addr function_input uint8 size=1; nbyte function_input uint8 size=1; reg function_input uint8 size=1; data function_input uint8 size=63; err function_output; data function_output; addr function_input uint8 size=1; nbyte function_input uint8 size=1; err function_output boolean; reg function_input uint8 size=1; write_buffer local uint8 size=63; read_err local boolean size=1; write_err local boolean size=1; read_buffer local uint8 size=64; raw_acc local int16 size=3; raw_gyro local int16 size=3; raw_temp local int16 size=1; raw_acc_calibrated output double size=3 =[0 0 -9.80665]; raw_gyro_calibrated output double size=3 =[0 0 0]; PAR_OFFSET_ACC parameter double size=3; PAR_OFFSET_GYRO parameter double size=3; PAR_SENS_ACC parameter double size=3; PAR_SENS_GYRO parameter double size=3; filter_reset output boolean

== matlab function cm_custom/SFB a2m map/M_a2m ==
  data: psi input; the1 output; the input; the2 output; par_r parameter size=1; par_w parameter size=1; par_yawMax parameter size=1; par_pitchMax parameter size=1
function [the1, the2] = fcn(psi, the, par_r, par_w, par_yawMax, par_pitchMax)

%% abs limits
if abs(psi) > par_yawMax
    psi = sign(psi) * par_yawMax;
end

if abs(the) > par_pitchMax
    the = sign(the) * par_pitchMax;
end

%% main
thep = the;
thef = asin( -par_w / (2 * par_r) * tan(psi));

the1 = thep + thef;
the2 = thep - thef;
